simulink model "msl_subsys_fcncall1"  (Simulink 8.0)
settings: Solver=FixedStepDiscrete  StartTime=0.0  StopTime=10.0  FixedStep=1  RelTol=1e-3
settings Model: Creator=The MathWorks Inc.  LastModifiedBy=skalmane  CovMetricSettings=d  ExtModeAutoUpdateStatusClock=off
settings DataIOCC: SignalLoggingSaveFormat=ModelDataLogs  SaveState=on
settings OptimizationCC: BlockReduction=off  BooleanDataType=off  InlineInvariantSignals=on  InitFltsAndDblsToZero=on  LifeSpan=1
settings DebuggingCC: SaveWithParameterizedLinksMsg=none  SignalResolutionControl=TryResolveAllWithWarning  SolverPrmCheckMsg=none  MultiTaskDSMMsg=warning  MultiTaskCondExecSysMsg=none  SigSpecEnsureSampleTimeMsg=none  FcnCallInpInsideContextMsg=UseLocalSettings  StrictBusMsg=None
settings SFSimCC: SimParseCustomCode=off
settings RTWCC: SystemTargetFile=ert.tlc  TemplateMakefile=ert_default_tmf  Description=Real-Time Workshop Embedded Coder (no auto configuration)  ProcessScript=ert_make_rtw_hook  IncludeERTFirstTime=on
settings CodeAppCC: IgnoreCustomStorageClasses=off
settings ERTTargetCC: TargetFcnLib=ansi_tfl_tmw.mat  CodeReplacementLibrary=ANSI_C  MultiwordLength=2048  GenerateSampleERTMain=on  InlinedParameterPlacement=NonHierarchical  ERTCustomFileTemplate=example_file_process.tlc  ConvertIfToSwitch=off  SuppressUnreachableDefaultCases=off

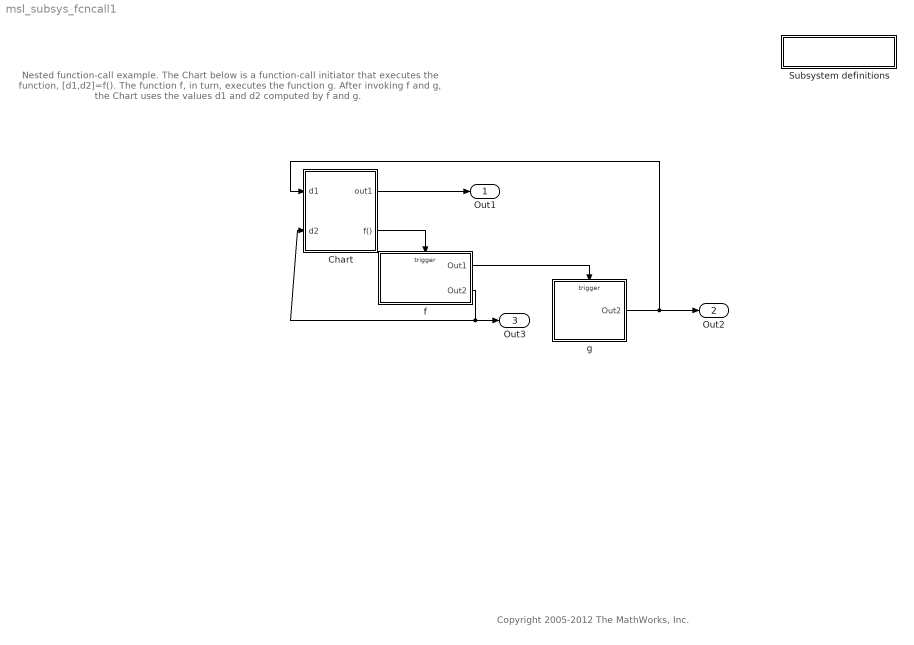
== system msl_subsys_fcncall1 ==
  note: Nested function-call example.
      |
      | The Chart below is a function-call initiator that executes the function, [d1,d2]=f().
      | The function f, in turn, executes the function g.
      | After invoking f and g, the Chart uses the values d1 and d2 computed by f and g.
  note: Copyright 2005-2012 The MathWorks, Inc.
  " Subsystem definitions" : Subsystem
      settings: OpenFcn=helpview(fullfile(docroot,'simulink','helptargets.map'),'subsystem_defs')
      mask Display: disp('Subsystem\ndefinitions')
  Chart : Stateflow chart  TreatAsAtomicUnit=on
  f : Subsystem  TreatAsAtomicUnit=on
  g : Subsystem  TreatAsAtomicUnit=on
  Out1 : Outport
  Out2 : Outport  Port=2
  Out3 : Outport  Port=3
      settings: OpenFcn=helpview(fullfile(docroot,'simulink','helptargets.map'),'subsystem_defs')
  wires:
  Chart/2(f()) -> f/Trigger
  f/1(Out1) -> g/Trigger
  f/2(Out2) -> Out3/1, Chart/2(d2)
  g/1(Out2) -> Out2/1, Chart/1(d1)
  Chart/1(out1) -> Out1/1

== system msl_subsys_fcncall1/ Subsystem definitions ==

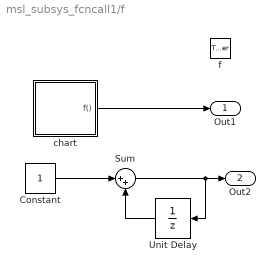
== system msl_subsys_fcncall1/f ==
  f : TriggerPort  TriggerType=function-call
  Constant : Constant
  Sum : Sum  Inputs=|++  SaturateOnIntegerOverflow=on  InputSameDT=on  OutDataTypeStr=Inherit: Same as first input
  Unit Delay : UnitDelay  SampleTime=-1
  chart : Stateflow chart  TreatAsAtomicUnit=on
  Out1 : Outport
  Out2 : Outport  Port=2
  wires:
  chart/1(f()) -> Out1/1
  Constant/1 -> Sum/1
  Unit Delay/1 -> Sum/2
  Sum/1 -> Out2/1, Unit Delay/1

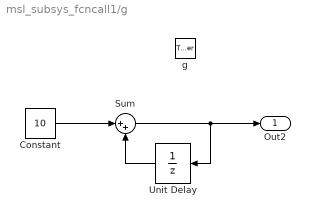
== system msl_subsys_fcncall1/g ==
  g : TriggerPort  TriggerType=function-call
  Constant : Constant  Value=10
  Sum : Sum  Inputs=|++  SaturateOnIntegerOverflow=on  InputSameDT=on  OutDataTypeStr=Inherit: Same as first input
  Unit Delay : UnitDelay  SampleTime=-1
  Out2 : Outport
  wires:
  Constant/1 -> Sum/1
  Unit Delay/1 -> Sum/2
  Sum/1 -> Out2/1, Unit Delay/1

== stateflow chart Chart ==
  state one/
    entry:f;out1=d1+d2;
  state two/
    entry: f;out1=d1-d2;
  (default) -> one
  one -> two
  two -> one
  data: d1 input double; d2 input double; out1 output double; out local double
  events: f output FUNCTION_CALL_EVENT

== stateflow chart f/chart ==
  state one/
    entry: f;
  state two/
    entry: f;
  one -> two
  (default) -> one
  two -> one
  events: f output FUNCTION_CALL_EVENT
